simulink model "SPGF_FSK_0000_R2019b"  (R2019b)
settings: Solver=ode3  SolverName=ode4  StartTime=0.0  StopTime=1.4  FixedStep=50e-6/50  RelTol=1e-3  EnableMultiTasking=on
undefined symbols (not defined in the file): D11, Delta
libraries: powerlib x2544, powerlib_meascontrol x204, simulink x24
(part 12 of 33)

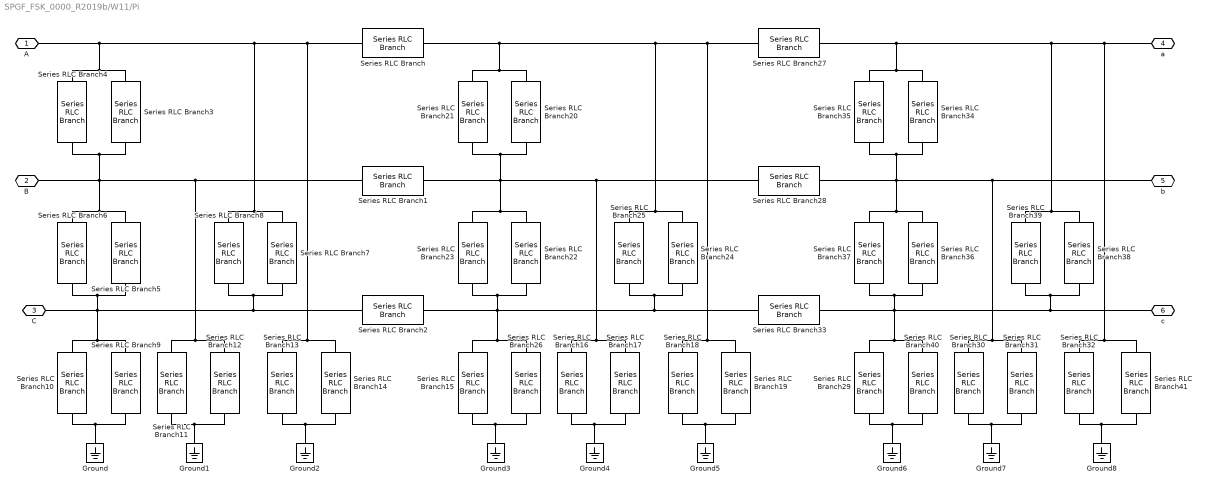
== system SPGF_FSK_0000_R2019b/W11/Pi ==
  Ground{,1..8} (9 alike) : powerlib/Elements/Ground  LConnTagsString=a
  Series RLC Branch{,1..2,27..28,33} (6 alike) : powerlib/Elements/Series RLC Branch  LConnTagsString=__new0  RConnTagsString=__new0  BranchType=RL  Resistance=R/2  Inductance=L/2  SetiL0=off  InitialCurrent=0  Capacitance=1e-6  Setx0=off  InitialVoltage=0  Measurements=None
  Series RLC Branch{10..11,13,29..30,32} (6 alike) : powerlib/Elements/Series RLC Branch  LConnTagsString=__new0  RConnTagsString=__new0  BranchType=R  Resistance=Rfg*4  Inductance=L/2  SetiL0=off  InitialCurrent=0  Capacitance=1e-6  Setx0=off  InitialVoltage=0  Measurements=None
  Series RLC Branch{9,12,14,31,40..41} (6 alike) : powerlib/Elements/Series RLC Branch  LConnTagsString=__new0  RConnTagsString=__new0  BranchType=C  Resistance=R/2  Inductance=L/2  SetiL0=off  InitialCurrent=0  Capacitance=Cfg*0.25  Setx0=off  InitialVoltage=0  Measurements=None
  Series RLC Branch15 : powerlib/Elements/Series RLC Branch  LConnTagsString=__new0  RConnTagsString=__new0  BranchType=R  Resistance=Rfg*2  Inductance=L/2  SetiL0=off  InitialCurrent=0  Capacitance=1e-6  Setx0=off  InitialVoltage=0  Measurements=None
  Series RLC Branch16 : powerlib/Elements/Series RLC Branch  LConnTagsString=__new0  RConnTagsString=__new0  BranchType=R  Resistance=Rfg*2  Inductance=L/2  SetiL0=off  InitialCurrent=0  Capacitance=1e-6  Setx0=off  InitialVoltage=0  Measurements=None
  Series RLC Branch17 : powerlib/Elements/Series RLC Branch  LConnTagsString=__new0  RConnTagsString=__new0  BranchType=C  Resistance=R/2  Inductance=L/2  SetiL0=off  InitialCurrent=0  Capacitance=Cfg*0.5  Setx0=off  InitialVoltage=0  Measurements=None
  Series RLC Branch18 : powerlib/Elements/Series RLC Branch  LConnTagsString=__new0  RConnTagsString=__new0  BranchType=R  Resistance=Rfg*2  Inductance=L/2  SetiL0=off  InitialCurrent=0  Capacitance=1e-6  Setx0=off  InitialVoltage=0  Measurements=None
  Series RLC Branch19 : powerlib/Elements/Series RLC Branch  LConnTagsString=__new0  RConnTagsString=__new0  BranchType=C  Resistance=R/2  Inductance=L/2  SetiL0=off  InitialCurrent=0  Capacitance=Cfg*0.5  Setx0=off  InitialVoltage=0  Measurements=None
  Series RLC Branch20 : powerlib/Elements/Series RLC Branch  LConnTagsString=__new0  RConnTagsString=__new0  BranchType=C  Resistance=R/2  Inductance=L/2  SetiL0=off  InitialCurrent=0  Capacitance=Cmf*0.5  Setx0=off  InitialVoltage=0  Measurements=None
  Series RLC Branch21 : powerlib/Elements/Series RLC Branch  LConnTagsString=__new0  RConnTagsString=__new0  BranchType=R  Resistance=Rmf*2  Inductance=L/2  SetiL0=off  InitialCurrent=0  Capacitance=1e-6  Setx0=off  InitialVoltage=0  Measurements=None
  Series RLC Branch22 : powerlib/Elements/Series RLC Branch  LConnTagsString=__new0  RConnTagsString=__new0  BranchType=C  Resistance=R/2  Inductance=L/2  SetiL0=off  InitialCurrent=0  Capacitance=Cmf*0.5  Setx0=off  InitialVoltage=0  Measurements=None
  Series RLC Branch23 : powerlib/Elements/Series RLC Branch  LConnTagsString=__new0  RConnTagsString=__new0  BranchType=R  Resistance=Rmf*2  Inductance=L/2  SetiL0=off  InitialCurrent=0  Capacitance=1e-6  Setx0=off  InitialVoltage=0  Measurements=None
  Series RLC Branch24 : powerlib/Elements/Series RLC Branch  LConnTagsString=__new0  RConnTagsString=__new0  BranchType=C  Resistance=R/2  Inductance=L/2  SetiL0=off  InitialCurrent=0  Capacitance=Cmf*0.5  Setx0=off  InitialVoltage=0  Measurements=None
  Series RLC Branch25 : powerlib/Elements/Series RLC Branch  LConnTagsString=__new0  RConnTagsString=__new0  BranchType=R  Resistance=Rmf*2  Inductance=L/2  SetiL0=off  InitialCurrent=0  Capacitance=1e-6  Setx0=off  InitialVoltage=0  Measurements=None
  Series RLC Branch26 : powerlib/Elements/Series RLC Branch  LConnTagsString=__new0  RConnTagsString=__new0  BranchType=C  Resistance=R/2  Inductance=L/2  SetiL0=off  InitialCurrent=0  Capacitance=Cfg*0.5  Setx0=off  InitialVoltage=0  Measurements=None
  Series RLC Branch{3,5,7,34,36,38} (6 alike) : powerlib/Elements/Series RLC Branch  LConnTagsString=__new0  RConnTagsString=__new0  BranchType=C  Resistance=R/2  Inductance=L/2  SetiL0=off  InitialCurrent=0  Capacitance=Cmf*0.25  Setx0=off  InitialVoltage=0  Measurements=None
  Series RLC Branch{4,6,8,35,37,39} (6 alike) : powerlib/Elements/Series RLC Branch  LConnTagsString=__new0  RConnTagsString=__new0  BranchType=R  Resistance=Rmf*4  Inductance=L/2  SetiL0=off  InitialCurrent=0  Capacitance=1e-6  Setx0=off  InitialVoltage=0  Measurements=None
  A : PMIOPort  Side=Left
  B : PMIOPort  Port=2  Side=Left
  C : PMIOPort  Port=3  Side=Left
  a : PMIOPort  Port=4  Side=Right
  b : PMIOPort  Port=5  Side=Right
  c : PMIOPort  Port=6  Side=Right
  connections:
  Series RLC Branch12/LConn1 -- Series RLC Branch11/LConn1 -- Series RLC Branch5/LConn1 -- Series RLC Branch6/LConn1 -- B/RConn1 -- Series RLC Branch4/RConn1 -- Series RLC Branch3/RConn1 -- Series RLC Branch1/LConn1
  Series RLC Branch13/LConn1 -- A/RConn1 -- Series RLC Branch4/LConn1 -- Series RLC Branch3/LConn1 -- Series RLC Branch7/LConn1 -- Series RLC Branch8/LConn1 -- Series RLC Branch/LConn1 -- Series RLC Branch14/LConn1
  Series RLC Branch9/LConn1 -- Series RLC Branch2/LConn1 -- Series RLC Branch8/RConn1 -- Series RLC Branch7/RConn1 -- C/RConn1 -- Series RLC Branch5/RConn1 -- Series RLC Branch6/RConn1 -- Series RLC Branch10/LConn1
  Series RLC Branch9/RConn1 -- Ground/LConn1 -- Series RLC Branch10/RConn1
  Series RLC Branch12/RConn1 -- Series RLC Branch11/RConn1 -- Ground1/LConn1
  Series RLC Branch13/RConn1 -- Series RLC Branch14/RConn1 -- Ground2/LConn1
  Series RLC Branch17/LConn1 -- Series RLC Branch16/LConn1 -- Series RLC Branch28/LConn1 -- Series RLC Branch1/RConn1 -- Series RLC Branch23/LConn1 -- Series RLC Branch22/LConn1 -- Series RLC Branch20/RConn1 -- Series RLC Branch21/RConn1
  Series RLC Branch21/LConn1 -- Series RLC Branch20/LConn1 -- Series RLC Branch/RConn1 -- Series RLC Branch27/LConn1 -- Series RLC Branch19/LConn1 -- Series RLC Branch18/LConn1 -- Series RLC Branch24/LConn1 -- Series RLC Branch25/LConn1
  Series RLC Branch26/LConn1 -- Series RLC Branch15/LConn1 -- Series RLC Branch2/RConn1 -- Series RLC Branch33/LConn1 -- Series RLC Branch25/RConn1 -- Series RLC Branch24/RConn1 -- Series RLC Branch22/RConn1 -- Series RLC Branch23/RConn1
  Series RLC Branch26/RConn1 -- Series RLC Branch15/RConn1 -- Ground3/LConn1
  Ground4/LConn1 -- Series RLC Branch17/RConn1 -- Series RLC Branch16/RConn1
  Ground5/LConn1 -- Series RLC Branch18/RConn1 -- Series RLC Branch19/RConn1
  Series RLC Branch31/LConn1 -- b/RConn1 -- Series RLC Branch35/RConn1 -- Series RLC Branch34/RConn1 -- Series RLC Branch36/LConn1 -- Series RLC Branch37/LConn1 -- Series RLC Branch28/RConn1 -- Series RLC Branch30/LConn1
  Series RLC Branch34/LConn1 -- a/RConn1 -- Series RLC Branch41/LConn1 -- Series RLC Branch32/LConn1 -- Series RLC Branch38/LConn1 -- Series RLC Branch39/LConn1 -- Series RLC Branch27/RConn1 -- Series RLC Branch35/LConn1
  Series RLC Branch29/LConn1 -- Series RLC Branch36/RConn1 -- Series RLC Branch37/RConn1 -- c/RConn1 -- Series RLC Branch39/RConn1 -- Series RLC Branch38/RConn1 -- Series RLC Branch33/RConn1 -- Series RLC Branch40/LConn1
  Series RLC Branch29/RConn1 -- Series RLC Branch40/RConn1 -- Ground6/LConn1
  Series RLC Branch31/RConn1 -- Series RLC Branch30/RConn1 -- Ground7/LConn1
  Series RLC Branch32/RConn1 -- Series RLC Branch41/RConn1 -- Ground8/LConn1

== system SPGF_FSK_0000_R2019b/W11/Q ==
  breaker : Subsystem  Commented=on  mask{SwitchA=on, SwitchB=on, SwitchC=on, InitialStatus=[0 0 0], BreakerResistance=0.0001, SnubberResistance=1e6, SnubberCapacitance=inf, TransitionTimes=[0.2], ShiftTimes=[0 0.02 0.04]}
      mask prompts: SwitchA "Switching of phase A"; SwitchB "Switching of phase B"; SwitchC "Switching of phase C"; InitialStatus "Initial status of phase breaker [A, B, C]"; BreakerResistance "Breaker resistance Ron (ohms) :"; SnubberResistance "Snubbers resistance Rp (ohms) :"; SnubberCapacitance "Snubbers capacitance Cp (F) :"; TransitionTimes "Transition times (s) :"; ShiftTimes "Time differences for switch [tA, tB, tC] (s) :"
      mask init: same as SPGF_FSK_0000_R2019b/Feed/Q/breaker
      mask Display:
      | % port_label('input',1,'Iabc');
      | 
      | port_label('lconn',1,'A');
      | port_label('lconn',2,'B');
      | port_label('lconn',3,'C');
      | 
      | port_label('rconn',1,'a');
      | port_label('rconn',2,'b');
      | port_label('rconn',3,'c');
      | 
      | disp('   Q    ');
  meas : Subsystem
  shunt : Subsystem
  A : PMIOPort  Side=Right
  B : PMIOPort  Port=2  Side=Right
  C : PMIOPort  Port=3  Side=Right
  a : PMIOPort  Port=4  Side=Left
  b : PMIOPort  Port=5  Side=Left
  c : PMIOPort  Port=6  Side=Left
  connections:
  shunt/LConn3 -- breaker/LConn3 -- C/RConn1
  shunt/LConn2 -- breaker/LConn2 -- B/RConn1
  A/RConn1 -- breaker/LConn1 -- shunt/LConn1
  meas/RConn1 -- a/RConn1
  meas/RConn2 -- b/RConn1
  meas/RConn3 -- c/RConn1
  breaker/RConn3 -- shunt/RConn3 -- meas/LConn3
  breaker/RConn2 -- shunt/RConn2 -- meas/LConn2
  breaker/RConn1 -- shunt/RConn1 -- meas/LConn1

== system SPGF_FSK_0000_R2019b/W11/concentrated ==
  Ccs/1 : powerlib/Elements/Series RLC Branch  LConnTagsString=__new0  RConnTagsString=__new0  BranchType=C  Resistance=190  Inductance=1e-3  SetiL0=off  InitialCurrent=0  Capacitance=-C_matrix(1,2)/2  Setx0=off  InitialVoltage=0  Measurements=None
  Ccs/2 : powerlib/Elements/Series RLC Branch  LConnTagsString=__new0  RConnTagsString=__new0  BranchType=C  Resistance=190  Inductance=1e-3  SetiL0=off  InitialCurrent=0  Capacitance=-C_matrix(1,2)/2  Setx0=off  InitialVoltage=0  Measurements=None
  Ccs2/1 : powerlib/Elements/Series RLC Branch  LConnTagsString=__new0  RConnTagsString=__new0  BranchType=C  Resistance=190  Inductance=1e-3  SetiL0=off  InitialCurrent=0  Capacitance=-C_matrix(3,4)/2  Setx0=off  InitialVoltage=0  Measurements=None
  Ccs2/2 : powerlib/Elements/Series RLC Branch  LConnTagsString=__new0  RConnTagsString=__new0  BranchType=C  Resistance=190  Inductance=1e-3  SetiL0=off  InitialCurrent=0  Capacitance=-C_matrix(3,4)/2  Setx0=off  InitialVoltage=0  Measurements=None
  Ccs2/3 : powerlib/Elements/Series RLC Branch  LConnTagsString=__new0  RConnTagsString=__new0  BranchType=R  Resistance=-Rg_matrix(3,4)*2  Inductance=1e-3  SetiL0=off  InitialCurrent=0  Capacitance=Rg_matrix(3,4)*2  Setx0=off  InitialVoltage=0  Measurements=None
  Ccs2/4 : powerlib/Elements/Series RLC Branch  LConnTagsString=__new0  RConnTagsString=__new0  BranchType=R  Resistance=-Rg_matrix(3,4)*2  Inductance=1e-3  SetiL0=off  InitialCurrent=0  Capacitance=Rg_matrix(3,4)*2  Setx0=off  InitialVoltage=0  Measurements=None
  Ccs3/1 : powerlib/Elements/Series RLC Branch  LConnTagsString=__new0  RConnTagsString=__new0  BranchType=C  Resistance=190  Inductance=1e-3  SetiL0=off  InitialCurrent=0  Capacitance=-C_matrix(5,6)/2  Setx0=off  InitialVoltage=0  Measurements=None
  Ccs3/2 : powerlib/Elements/Series RLC Branch  LConnTagsString=__new0  RConnTagsString=__new0  BranchType=C  Resistance=190  Inductance=1e-3  SetiL0=off  InitialCurrent=0  Capacitance=-C_matrix(5,6)/2  Setx0=off  InitialVoltage=0  Measurements=None
  Ccs3/3 : powerlib/Elements/Series RLC Branch  LConnTagsString=__new0  RConnTagsString=__new0  BranchType=R  Resistance=-Rg_matrix(5,6)*2  Inductance=1e-3  SetiL0=off  InitialCurrent=0  Capacitance=-C_matrix(5,6)/2  Setx0=off  InitialVoltage=0  Measurements=None
  Ccs3/4 : powerlib/Elements/Series RLC Branch  LConnTagsString=__new0  RConnTagsString=__new0  BranchType=R  Resistance=-Rg_matrix(5,6)*2  Inductance=1e-3  SetiL0=off  InitialCurrent=0  Capacitance=-C_matrix(5,6)/2  Setx0=off  InitialVoltage=0  Measurements=None
  Csg/2 : powerlib/Elements/Series RLC Branch  LConnTagsString=__new0  RConnTagsString=__new0  BranchType=C  Resistance=190  Inductance=1e-3  SetiL0=off  InitialCurrent=0  Capacitance=( C_matrix(1,2) + C_matrix(2,2) )/2  Setx0=off  InitialVoltage=0  Measurements=None
  Csg1/1 : powerlib/Elements/Series RLC Branch  LConnTagsString=__new0  RConnTagsString=__new0  BranchType=C  Resistance=190  Inductance=1e-3  SetiL0=off  InitialCurrent=0  Capacitance=( C_matrix(1,2) + C_matrix(2,2) )/2  Setx0=off  InitialVoltage=0  Measurements=None
  Csg2/1 : powerlib/Elements/Series RLC Branch  LConnTagsString=__new0  RConnTagsString=__new0  BranchType=C  Resistance=190  Inductance=1e-3  SetiL0=off  InitialCurrent=0  Capacitance=( C_matrix(3,4) + C_matrix(4,4) )/2  Setx0=off  InitialVoltage=0  Measurements=None
  Csg2/2 : powerlib/Elements/Series RLC Branch  LConnTagsString=__new0  RConnTagsString=__new0  BranchType=C  Resistance=190  Inductance=1e-3  SetiL0=off  InitialCurrent=0  Capacitance=( C_matrix(3,4) + C_matrix(4,4) )/2  Setx0=off  InitialVoltage=0  Measurements=None
  Csg3/1 : powerlib/Elements/Series RLC Branch  LConnTagsString=__new0  RConnTagsString=__new0  BranchType=C  Resistance=190  Inductance=1e-3  SetiL0=off  InitialCurrent=0  Capacitance=( C_matrix(5,6) + C_matrix(6,6) ) /2  Setx0=off  InitialVoltage=0  Measurements=None
  Csg3/2 : powerlib/Elements/Series RLC Branch  LConnTagsString=__new0  RConnTagsString=__new0  BranchType=C  Resistance=190  Inductance=1e-3  SetiL0=off  InitialCurrent=0  Capacitance=( C_matrix(5,6) + C_matrix(6,6) ) /2  Setx0=off  InitialVoltage=0  Measurements=None
  Ground{1..4} (4 alike) : powerlib/Elements/Ground  LConnTagsString=a
  RL : powerlib/Elements/Mutual Inductance  LConnTagsString=a|b|c|L4|L5|L6  RConnTagsString=A|B|C|R4|R5|R6  TypeOfMutual=Generalized mutual inductance  NumberOfWindings=6  SelfImpedance1=[1.1 1.1e-03]  SelfImpedance2=[ 1.1 1.1e-03]  ThreeWindings=on  SelfImpedance3=[ 1.1 1.1e-03]  MutualImpedance=[1.0 1.0e-03]  InductanceMatrix=L_matrix  ResistanceMatrix=R_matrix  Measurements=None
      settings: AttributesFormatString=\n
  Rcs*2 : powerlib/Elements/Series RLC Branch  LConnTagsString=__new0  RConnTagsString=__new0  BranchType=R  Resistance=-Rg_matrix(1,2)*2  Inductance=1e-3  SetiL0=off  InitialCurrent=0  Capacitance=Rg_matrix(1,2)*2  Setx0=off  InitialVoltage=0  Measurements=None
  Rgcs1/1 : powerlib/Elements/Series RLC Branch  LConnTagsString=__new0  RConnTagsString=__new0  BranchType=R  Resistance=-Rg_matrix(1,2)*2  Inductance=1e-3  SetiL0=off  InitialCurrent=0  Capacitance=Rg_matrix(1,2)*2  Setx0=off  InitialVoltage=0  Measurements=None
  Rgsg1/1 : powerlib/Elements/Series RLC Branch  LConnTagsString=__new0  RConnTagsString=__new0  BranchType=R  Resistance=(Rg_matrix(4,4)+Rg_matrix(3,4))*2  Inductance=1e-3  SetiL0=off  InitialCurrent=0  Capacitance=Rg_matrix(1,2)*2  Setx0=off  InitialVoltage=0  Measurements=None
  Rgsg1/2 : powerlib/Elements/Series RLC Branch  LConnTagsString=__new0  RConnTagsString=__new0  BranchType=R  Resistance=(Rg_matrix(2,2)+Rg_matrix(1,2))*2  Inductance=1e-3  SetiL0=off  InitialCurrent=0  Capacitance=Rg_matrix(1,2)*2  Setx0=off  InitialVoltage=0  Measurements=None
  Rgsg1/3 : powerlib/Elements/Series RLC Branch  LConnTagsString=__new0  RConnTagsString=__new0  BranchType=R  Resistance=(Rg_matrix(4,4)+Rg_matrix(3,4))*2  Inductance=1e-3  SetiL0=off  InitialCurrent=0  Capacitance=Rg_matrix(1,2)*2  Setx0=off  InitialVoltage=0  Measurements=None
  Rgsg1/4 : powerlib/Elements/Series RLC Branch  LConnTagsString=__new0  RConnTagsString=__new0  BranchType=R  Resistance=(Rg_matrix(2,2)+Rg_matrix(1,2))*2  Inductance=1e-3  SetiL0=off  InitialCurrent=0  Capacitance=Rg_matrix(1,2)*2  Setx0=off  InitialVoltage=0  Measurements=None
  Rsg*2 : powerlib/Elements/Series RLC Branch  LConnTagsString=__new0  RConnTagsString=__new0  BranchType=R  Resistance=(Rg_matrix(6,6)+Rg_matrix(5,6))*2  Inductance=1e-3  SetiL0=off  InitialCurrent=0  Capacitance=Rg_matrix(1,2)*2  Setx0=off  InitialVoltage=0  Measurements=None
  Rsg1/1 : powerlib/Elements/Series RLC Branch  LConnTagsString=__new0  RConnTagsString=__new0  BranchType=R  Resistance=(Rg_matrix(6,6)+Rg_matrix(5,6))*2  Inductance=1e-3  SetiL0=off  InitialCurrent=0  Capacitance=Rg_matrix(1,2)*2  Setx0=off  InitialVoltage=0  Measurements=None
  A : PMIOPort  Side=Left
  B : PMIOPort  Port=2  Side=Left
  C : PMIOPort  Port=3  Side=Left
  a : PMIOPort  Port=4  Side=Right
  b : PMIOPort  Port=5  Side=Right
  c : PMIOPort  Port=6  Side=Right
  connections:
  RL/LConn5 -- Ccs3/2/RConn1 -- Ccs3/3/RConn1 -- C/RConn1
  RL/LConn3 -- Ccs2/2/RConn1 -- Ccs2/3/RConn1 -- B/RConn1
  RL/LConn1 -- Ccs/2/RConn1 -- Rcs*2/RConn1 -- A/RConn1
  RL/RConn5 -- Ccs3/1/RConn1 -- Ccs3/4/RConn1 -- c/RConn1
  RL/RConn3 -- Ccs2/1/RConn1 -- Ccs2/4/RConn1 -- b/RConn1
  RL/RConn1 -- Ccs/1/RConn1 -- Rgcs1/1/RConn1 -- a/RConn1
  Csg/2/RConn1 -- Ground1/LConn1 -- Csg3/2/RConn1 -- Rgsg1/2/RConn1 -- Rgsg1/1/RConn1 -- Rsg*2/RConn1 -- Csg2/2/RConn1
  Ccs3/4/LConn1 -- Ccs3/1/LConn1 -- RL/RConn6 -- RL/RConn2 -- Csg1/1/LConn1 -- Rgcs1/1/LConn1 -- Rgsg1/4/LConn1 -- Ccs/1/LConn1 -- RL/RConn4 -- Ccs2/1/LConn1 -- Csg2/1/LConn1 -- Ccs2/4/LConn1 -- Rgsg1/3/LConn1 -- Ground4/LConn1 -- Rsg1/1/LConn1 -- Csg3/1/LConn1
  Csg1/1/RConn1 -- Ground2/LConn1 -- Csg3/1/RConn1 -- Rgsg1/4/RConn1 -- Rgsg1/3/RConn1 -- Rsg1/1/RConn1 -- Csg2/1/RConn1
  RL/LConn2 -- Ccs/2/LConn1 -- Rcs*2/LConn1 -- Csg/2/LConn1 -- Rgsg1/2/LConn1 -- Ccs2/2/LConn1 -- Ccs2/3/LConn1 -- Csg2/2/LConn1 -- Rgsg1/1/LConn1 -- RL/LConn4 -- Ground3/LConn1 -- Ccs3/2/LConn1 -- Ccs3/3/LConn1 -- Csg3/2/LConn1 -- Rsg*2/LConn1 -- RL/LConn6

== system SPGF_FSK_0000_R2019b/W12/DPL ==
  Ccs2/1 : powerlib/Elements/Series RLC Branch  LConnTagsString=__new0  RConnTagsString=__new0  BranchType=R  Resistance=-Rg_matrix(3,4)*2  Inductance=1e-3  SetiL0=off  InitialCurrent=0  Capacitance=Rg_matrix(3,4)*2  Setx0=off  InitialVoltage=0  Measurements=None
  Ccs2/3 : powerlib/Elements/Series RLC Branch  LConnTagsString=__new0  RConnTagsString=__new0  BranchType=R  Resistance=-Rg_matrix(3,4)*2  Inductance=1e-3  SetiL0=off  InitialCurrent=0  Capacitance=Rg_matrix(3,4)*2  Setx0=off  InitialVoltage=0  Measurements=None
  Ccs3/1 : powerlib/Elements/Series RLC Branch  LConnTagsString=__new0  RConnTagsString=__new0  BranchType=R  Resistance=-Rg_matrix(5,6)*2  Inductance=1e-3  SetiL0=off  InitialCurrent=0  Capacitance=-C_matrix(5,6)/2  Setx0=off  InitialVoltage=0  Measurements=None
  Ccs3/3 : powerlib/Elements/Series RLC Branch  LConnTagsString=__new0  RConnTagsString=__new0  BranchType=R  Resistance=-Rg_matrix(5,6)*2  Inductance=1e-3  SetiL0=off  InitialCurrent=0  Capacitance=-C_matrix(5,6)/2  Setx0=off  InitialVoltage=0  Measurements=None
  DPL : powerlib/Elements/Distributed Parameters Line  Phases=6  Length=LineLength  Frequency=Frequency  Resistance=R_matrix  Inductance=L_matrix  Capacitance=C_matrix  x1=[-5.3e-05 -1.50939355674186 0 0 0 0 -8872.61351094603;-5.25e-05 -1.50980377797187 0 0 0 0 -8871.84731916744;-5.2e-05 -1.51021396194896 0 0 0 0 -8871.0809084848;-5.15e-05 -1.51062410866302 0 0 0 0 -8870.314278917;-5.1e-05 -1.51103421810392 0 0 0 0 -8869.54743048298;-5.05e-05 -1.51144429026155 0 0 0 0 -8868.78036320164;-5e-05 -1.51185432512578 0 0 0 0 -8868.01307709192;-4.95e-05 -1.51226432268651 0 0 0 0 -8867.24557217275;-4.9e-05 -1.5126742829336 0 0 0 0 -8866.47784846306;-4.85e-05 -1.51308420585696 0 0 0 0 -8865.70990598181;-4.8e-05 -1.51349409144646 0 0 0 0 -8864.94174474793;-4.75e-05 -1.51390393969199 0 0 0 0 -8864.17336478037;-4.7e-05 -1.51431375058343 0 0 0 0 -8863.40476609811;-4.65e-05 -1.51472352411069 0 0 0 0 -8862.63594872011;-4.6e-05 -1.51513326026364 0 0 0 0 -8861.86691266532;-4.55e-05 -1.51554295903217 0 0 0 0 -8861.09765795274;-4.5e-05 -1.51595262040618 0 0 0 0 -8860.32818460133;-4.45e-05 -1.51636224437556 0 0 0 0 -8859.55849263009;-4.4e-05 -1.5167718309302 0 0 0 0 -8858.78858205801;-4.35e-05 -1.51718138005999 0 0 0 0 -8858.01845290408;-4.3e-05 -1.51759089175484 0 0 0 0 -8857.2481051873;-4.25e-05 -1.51800036600463 0 0 0 0 -8856.47753892669;-4.2e-05 -1.51840980279926 0 0 0 0 -8855.70675414126;-4.15e-05 -1.51881920212864 0 0 0 0 -8854.93575085002;-4.1e-05 -1.51922856398265 0 0 0 0 -8854.164529072;-4.05e-05 -1.5196378883512 0 0 0 0 -8853.39308882622;-4e-05 -1.52004717522418 0 0 0 0 -8852.62143013173;-3.95e-05 -1.52045642459151 0 0 0 0 -8851.84955300756;-3.9e-05 -1.52086563644308 0 0 0 0 -8851.07745747275;-3.85e-05 -1.52127481076879 0 0 0 0 -8850.30514354637;-3.8e-05 -1.52168394755855 0 0 0 0 -8849.53261124746;-3.75e-05 -1.52209304680227 0 0 0 0 -8848.75986059508;-3.7e-05 -1.52250210848984 0 0 0 0 -8847.9868916083;-3.65e-05 -1.52291113261118 0 0 0 0 -8847.2137043062;-3.6e-05 -1.5233201191562 0 0 0 0 -8846.44029870786;-3.55e-05 -1.5237290681148 0 0 0 0 -8845.66667483234;-3.5e-05 -1.52413797947689 0 0 0 0 -8844.89283269876;-3.45e-05 -1.52454685323238 0 0 0 0 -8844.11877232619;-3.4e-05 -1.52495568937119 0 0 0 0 -8843.34449373373;-3.35e-05 -1.52536448788322 0 0 0 0 -8842.5699969405;-3.3e-05 -1.52577324875839 0 0 0 0 -8841.79528196559;-3.25e-05 -1.52618197198662 0 0 0 0 -8841.02034882814;-3.2e-05 -1.52659065755782 0 0 0 0 -8840.24519754725;-3.15e-05 -1.5269993054619 0 0 0 0 -8839.46982814205;-3.1e-05 -1.52740791568878 0 0 0 0 -8838.69424063168;-3.05e-05 -1.52781648822839 0 0 0 0 -8837.91843503527;-3e-05 -1.52822502307063 0 0 0 0 -8837.14241137197;-2.95e-05 -1.52863352020544 0 0 0 0 -8836.36616966091;-2.9e-05 -1.52904197962272 0 0 0 0 -8835.58970992126;-2.85e-05 -1.52945040131241 0 0 0 0 -8834.81303217217;-2.8e-05 -1.52985878526441 0 0 0 0 -8834.03613643281;-2.75e-05 -1.53026713146867 0 0 0 0 -8833.25902272235;-2.7e-05 -1.5306754399151 0 0 0 0 -8832.48169105995;-2.65e-05 -1.53108371059362 0 0 0 0 -8831.70414146481;-2.6e-05 -1.53149194349417 0 0 0 0 -8830.9263739561;-2.55e-05 -1.53190013860667 0 0 0 0 -8830.14838855301;-2.5e-05 -1.53230829592105 0 0 0 0 -8829.37018527475;-2.45e-05 -1.53271641542724 0 0 0 0 -8828.59176414051;-2.4e-05 -1.53312449711517 0 0 0 0 -8827.8131251695;-2.35e-05 -1.53353254097476 0 0 0 0 -8827.03426838094;-2.3e-05 -1.53394054699596 0 0 0 0 -8826.25519379403;-2.25e-05 -1.53434851516869 0 0 0 0 -8825.475901428;-2.2e-05 -1.53475644548289 0 0 0 0 -8824.69639130209;-2.15e-05 -1.53516433792849 0 0 0 0 -8823.91666343552;-2.1e-05 -1.53557219249543 0 0 0 0 -8823.13671784754;-2.05e-05 -1.53598000917365 0 0 0 0 -8822.35655455738;-2e-05 -1.53638778795308 0 0 0 0 -8821.5761735843;-1.95e-05 -1.53679552882365 0 0 0 0 -8820.79557494756;-1.9e-05 -1.53720323177532 0 0 0 0 -8820.0147586664;-1.85e-05 -1.53761089679802 0 0 0 0 -8819.23372476011;-1.8e-05 -1.53801852388169 0 0 0 0 -8818.45247324795;-1.75e-05 -1.53842611301628 0 0 0 0 -8817.67100414919;-1.7e-05 -1.53883366419172 0 0 0 0 -8816.88931748313;-1.65e-05 -1.53924117739797 0 0 0 0 -8816.10741326904;-1.6e-05 -1.53964865262496 0 0 0 0 -8815.32529152621;-1.55e-05 ...(+2780 chars)]  x2=[-5.3e-05 -1.50564703819446 0 0 0 0 -8948.23948235752;-5.25e-05 -1.50606747011388 0 0 0 0 -8947.47202642379;-5.2e-05 -1.50648786487257 0 0 0 0 -8946.70434972004;-5.15e-05 -1.50690822246016 0 0 0 0 -8945.93645226522;-5.1e-05 -1.50732854286628 0 0 0 0 -8945.16833407825;-5.05e-05 -1.50774882608056 0 0 0 0 -8944.39999517811;-5e-05 -1.50816907209263 0 0 0 0 -8943.63143558374;-4.95e-05 -1.50858928089212 0 0 0 0 -8942.86265531411;-4.9e-05 -1.50900945246867 0 0 0 0 -8942.09365438819;-4.85e-05 -1.50942958681189 0 0 0 0 -8941.32443282496;-4.8e-05 -1.50984968391144 0 0 0 0 -8940.55499064338;-4.75e-05 -1.51026974375693 0 0 0 0 -8939.78532786246;-4.7e-05 -1.51068976633802 0 0 0 0 -8939.01544450117;-4.65e-05 -1.51110975164433 0 0 0 0 -8938.24534057852;-4.6e-05 -1.5115296996655 0 0 0 0 -8937.47501611351;-4.55e-05 -1.51194961039117 0 0 0 0 -8936.70447112514;-4.5e-05 -1.51236948381097 0 0 0 0 -8935.93370563242;-4.45e-05 -1.51278931991456 0 0 0 0 -8935.16271965438;-4.4e-05 -1.51320911869157 0 0 0 0 -8934.39151321004;-4.35e-05 -1.51362888013164 0 0 0 0 -8933.62008631842;-4.3e-05 -1.51404860422441 0 0 0 0 -8932.84843899856;-4.25e-05 -1.51446829095953 0 0 0 0 -8932.0765712695;-4.2e-05 -1.51488794032664 0 0 0 0 -8931.30448315029;-4.15e-05 -1.5153075523154 0 0 0 0 -8930.53217465997;-4.1e-05 -1.51572712691543 0 0 0 0 -8929.75964581761;-4.05e-05 -1.5161466641164 0 0 0 0 -8928.98689664226;-4e-05 -1.51656616390795 0 0 0 0 -8928.21392715298;-3.95e-05 -1.51698562627973 0 0 0 0 -8927.44073736886;-3.9e-05 -1.51740505122139 0 0 0 0 -8926.66732730897;-3.85e-05 -1.51782443872258 0 0 0 0 -8925.89369699239;-3.8e-05 -1.51824378877296 0 0 0 0 -8925.11984643821;-3.75e-05 -1.51866310136217 0 0 0 0 -8924.34577566553;-3.7e-05 -1.51908237647987 0 0 0 0 -8923.57148469344;-3.65e-05 -1.51950161411571 0 0 0 0 -8922.79697354105;-3.6e-05 -1.51992081425936 0 0 0 0 -8922.02224222747;-3.55e-05 -1.52033997690046 0 0 0 0 -8921.24729077181;-3.5e-05 -1.52075910202868 0 0 0 0 -8920.4721191932;-3.45e-05 -1.52117818963367 0 0 0 0 -8919.69672751077;-3.4e-05 -1.52159723970509 0 0 0 0 -8918.92111574364;-3.35e-05 -1.52201625223261 0 0 0 0 -8918.14528391096;-3.3e-05 -1.52243522720588 0 0 0 0 -8917.36923203185;-3.25e-05 -1.52285416461457 0 0 0 0 -8916.59296012548;-3.2e-05 -1.52327306444834 0 0 0 0 -8915.81646821101;-3.15e-05 -1.52369192669685 0 0 0 0 -8915.03975630757;-3.1e-05 -1.52411075134977 0 0 0 0 -8914.26282443435;-3.05e-05 -1.52452953839676 0 0 0 0 -8913.48567261051;-3e-05 -1.5249482878275 0 0 0 0 -8912.70830085523;-2.95e-05 -1.52536699963164 0 0 0 0 -8911.93070918768;-2.9e-05 -1.52578567379886 0 0 0 0 -8911.15289762706;-2.85e-05 -1.52620431031883 0 0 0 0 -8910.37486619256;-2.8e-05 -1.52662290918122 0 0 0 0 -8909.59661490336;-2.75e-05 -1.5270414703757 0 0 0 0 -8908.81814377869;-2.7e-05 -1.52745999389194 0 0 0 0 -8908.03945283773;-2.65e-05 -1.52787847971962 0 0 0 0 -8907.26054209972;-2.6e-05 -1.5282969278484 0 0 0 0 -8906.48141158386;-2.55e-05 -1.52871533826797 0 0 0 0 -8905.70206130938;-2.5e-05 -1.529133710968 0 0 0 0 -8904.92249129551;-2.45e-05 -1.52955204593817 0 0 0 0 -8904.14270156148;-2.4e-05 -1.52997034316816 0 0 0 0 -8903.36269212654;-2.35e-05 -1.53038860264764 0 0 0 0 -8902.58246300993;-2.3e-05 -1.53080682436629 0 0 0 0 -8901.80201423091;-2.25e-05 -1.5312250083138 0 0 0 0 -8901.02134580872;-2.2e-05 -1.53164315447985 0 0 0 0 -8900.24045776264;-2.15e-05 -1.53206126285412 0 0 0 0 -8899.45935011192;-2.1e-05 -1.53247933342629 0 0 0 0 -8898.67802287585;-2.05e-05 -1.53289736618605 0 0 0 0 -8897.8964760737;-2e-05 -1.53331536112309 0 0 0 0 -8897.11470972475;-1.95e-05 -1.53373331822708 0 0 0 0 -8896.3327238483;-1.9e-05 -1.53415123748772 0 0 0 0 -8895.55051846364;-1.85e-05 -1.5345691188947 0 0 0 0 -8894.76809359006;-1.8e-05 -1.5349869624377 0 0 0 0 -8893.98544924688;-1.75e-05 -1.53540476810641 0 0 0 0 -8893.20258545341;-1.7e-05 -1.53582253589054 0 0 0 0 -8892.41950222896;-1.65e-05 -1.53624026577976 0 0 0 0 -8891.63619959285;-1.6e-05 -1.53665795776377 0 0 0 0 -8890.85267756441;-1.55e-05 ...(+2786 chars)]  x3=[-5.3e-05 0.0131139201948921 0 0 0 0 -275.39648268413;-5.25e-05 0.0131100972254946 0 0 0 0 -275.39032083345;-5.2e-05 0.0131062739326184 0 0 0 0 -275.384152187786;-5.15e-05 0.0131024503163578 0 0 0 0 -275.37797674729;-5.1e-05 0.0130986263768073 0 0 0 0 -275.371794512115;-5.05e-05 0.013094802114061 0 0 0 0 -275.365605482414;-5e-05 0.0130909775282135 0 0 0 0 -275.359409658338;-4.95e-05 0.0130871526193591 0 0 0 0 -275.353207040042;-4.9e-05 0.0130833273875921 0 0 0 0 -275.346997627677;-4.85e-05 0.013079501833007 0 0 0 0 -275.340781421397;-4.8e-05 0.0130756759556981 0 0 0 0 -275.334558421356;-4.75e-05 0.0130718497557598 0 0 0 0 -275.328328627708;-4.7e-05 0.0130680232332866 0 0 0 0 -275.322092040605;-4.65e-05 0.0130641963883728 0 0 0 0 -275.315848660201;-4.6e-05 0.0130603692211129 0 0 0 0 -275.309598486652;-4.55e-05 0.0130565417316013 0 0 0 0 -275.30334152011;-4.5e-05 0.0130527139199324 0 0 0 0 -275.297077760731;-4.45e-05 0.0130488857862007 0 0 0 0 -275.290807208668;-4.4e-05 0.0130450573305007 0 0 0 0 -275.284529864077;-4.35e-05 0.0130412285529268 0 0 0 0 -275.278245727113;-4.3e-05 0.0130373994535735 0 0 0 0 -275.27195479793;-4.25e-05 0.0130335700325352 0 0 0 0 -275.265657076684;-4.2e-05 0.0130297402899065 0 0 0 0 -275.25935256353;-4.15e-05 0.0130259102257818 0 0 0 0 -275.253041258624;-4.1e-05 0.0130220798402557 0 0 0 0 -275.246723162122;-4.05e-05 0.0130182491334227 0 0 0 0 -275.240398274178;-4e-05 0.0130144181053772 0 0 0 0 -275.23406659495;-3.95e-05 0.0130105867562138 0 0 0 0 -275.227728124594;-3.9e-05 0.0130067550860271 0 0 0 0 -275.221382863266;-3.85e-05 0.0130029230949115 0 0 0 0 -275.215030811122;-3.8e-05 0.0129990907829617 0 0 0 0 -275.20867196832;-3.75e-05 0.0129952581502722 0 0 0 0 -275.202306335015;-3.7e-05 0.0129914251969375 0 0 0 0 -275.195933911367;-3.65e-05 0.0129875919230523 0 0 0 0 -275.18955469753;-3.6e-05 0.0129837583287111 0 0 0 0 -275.183168693664;-3.55e-05 0.0129799244140084 0 0 0 0 -275.176775899925;-3.5e-05 0.012976090179039 0 0 0 0 -275.170376316471;-3.45e-05 0.0129722556238974 0 0 0 0 -275.16396994346;-3.4e-05 0.0129684207486782 0 0 0 0 -275.157556781051;-3.35e-05 0.0129645855534761 0 0 0 0 -275.151136829401;-3.3e-05 0.0129607500383856 0 0 0 0 -275.144710088668;-3.25e-05 0.0129569142035015 0 0 0 0 -275.138276559013;-3.2e-05 0.0129530780489183 0 0 0 0 -275.131836240592;-3.15e-05 0.0129492415747307 0 0 0 0 -275.125389133566;-3.1e-05 0.0129454047810334 0 0 0 0 -275.118935238092;-3.05e-05 0.012941567667921 0 0 0 0 -275.112474554331;-3e-05 0.0129377302354883 0 0 0 0 -275.106007082442;-2.95e-05 0.0129338924838298 0 0 0 0 -275.099532822584;-2.9e-05 0.0129300544130404 0 0 0 0 -275.093051774917;-2.85e-05 0.0129262160232146 0 0 0 0 -275.086563939601;-2.8e-05 0.0129223773144473 0 0 0 0 -275.080069316797;-2.75e-05 0.012918538286833 0 0 0 0 -275.073567906663;-2.7e-05 0.0129146989404666 0 0 0 0 -275.067059709362;-2.65e-05 0.0129108592754428 0 0 0 0 -275.060544725053;-2.6e-05 0.0129070192918563 0 0 0 0 -275.054022953897;-2.55e-05 0.0129031789898019 0 0 0 0 -275.047494396055;-2.5e-05 0.0128993383693743 0 0 0 0 -275.040959051688;-2.45e-05 0.0128954974306682 0 0 0 0 -275.034416920957;-2.4e-05 0.0128916561737786 0 0 0 0 -275.027868004024;-2.35e-05 0.0128878145988 0 0 0 0 -275.021312301051;-2.3e-05 0.0128839727058274 0 0 0 0 -275.014749812199;-2.25e-05 0.0128801304949555 0 0 0 0 -275.008180537629;-2.2e-05 0.0128762879662791 0 0 0 0 -275.001604477505;-2.15e-05 0.0128724451198931 0 0 0 0 -274.995021631989;-2.1e-05 0.0128686019558922 0 0 0 0 -274.988432001242;-2.05e-05 0.0128647584743712 0 0 0 0 -274.981835585427;-2e-05 0.0128609146754251 0 0 0 0 -274.975232384708;-1.95e-05 0.0128570705591486 0 0 0 0 -274.968622399247;-1.9e-05 0.0128532261256367 0 0 0 0 -274.962005629207;-1.85e-05 0.0128493813749841 0 0 0 0 -274.955382074751;-1.8e-05 0.0128455363072857 0 0 0 0 -274.948751736044;-1.75e-05 0.0128416909226364 0 0 0 0 -274.942114613248;-1.7e-05 0.0128378452211311 0 0 0 0 -274.935470706527;-1.65e-05 0.0128339992028646 0 0 0 0 ...(+2915 chars)]  x4=[-5.3e-05 -0.0324808035916861 0 0 0 0 14.9886458211936;-5.25e-05 -0.0324824208637865 0 0 0 0 15.004831786322;-5.2e-05 -0.0324840373344152 0 0 0 0 15.021017381221;-5.15e-05 -0.0324856530035325 0 0 0 0 15.0372026054913;-5.1e-05 -0.0324872678710983 0 0 0 0 15.0533874587335;-5.05e-05 -0.032488881937073 0 0 0 0 15.0695719405482;-5e-05 -0.0324904952014167 0 0 0 0 15.0857560505362;-4.95e-05 -0.0324921076640895 0 0 0 0 15.101939788298;-4.9e-05 -0.0324937193250517 0 0 0 0 15.1181231534344;-4.85e-05 -0.0324953301842635 0 0 0 0 15.1343061455461;-4.8e-05 -0.0324969402416852 0 0 0 0 15.1504887642338;-4.75e-05 -0.032498549497277 0 0 0 0 15.1666710090981;-4.7e-05 -0.0325001579509993 0 0 0 0 15.1828528797398;-4.65e-05 -0.0325017656028123 0 0 0 0 15.1990343757596;-4.6e-05 -0.0325033724526763 0 0 0 0 15.2152154967583;-4.55e-05 -0.0325049785005519 0 0 0 0 15.2313962423366;-4.5e-05 -0.0325065837463992 0 0 0 0 15.2475766120953;-4.45e-05 -0.0325081881901787 0 0 0 0 15.2637566056351;-4.4e-05 -0.0325097918318508 0 0 0 0 15.2799362225568;-4.35e-05 -0.032511394671376 0 0 0 0 15.2961154624612;-4.3e-05 -0.0325129967087146 0 0 0 0 15.312294324949;-4.25e-05 -0.0325145979438273 0 0 0 0 15.3284728096212;-4.2e-05 -0.0325161983766743 0 0 0 0 15.3446509160784;-4.15e-05 -0.0325177980072164 0 0 0 0 15.3608286439216;-4.1e-05 -0.0325193968354139 0 0 0 0 15.3770059927515;-4.05e-05 -0.0325209948612275 0 0 0 0 15.3931829621689;-4e-05 -0.0325225920846177 0 0 0 0 15.4093595517749;-3.95e-05 -0.0325241885055451 0 0 0 0 15.4255357611701;-3.9e-05 -0.0325257841239703 0 0 0 0 15.4417115899554;-3.85e-05 -0.0325273789398539 0 0 0 0 15.4578870377318;-3.8e-05 -0.0325289729531567 0 0 0 0 15.4740621041002;-3.75e-05 -0.0325305661638392 0 0 0 0 15.4902367886613;-3.7e-05 -0.0325321585718622 0 0 0 0 15.5064110910162;-3.65e-05 -0.0325337501771864 0 0 0 0 15.5225850107658;-3.6e-05 -0.0325353409797724 0 0 0 0 15.5387585475109;-3.55e-05 -0.0325369309795811 0 0 0 0 15.5549317008525;-3.5e-05 -0.0325385201765732 0 0 0 0 15.5711044703915;-3.45e-05 -0.0325401085707094 0 0 0 0 15.5872768557289;-3.4e-05 -0.0325416961619507 0 0 0 0 15.6034488564657;-3.35e-05 -0.0325432829502578 0 0 0 0 15.6196204722029;-3.3e-05 -0.0325448689355916 0 0 0 0 15.6357917025413;-3.25e-05 -0.032546454117913 0 0 0 0 15.6519625470821;-3.2e-05 -0.0325480384971828 0 0 0 0 15.6681330054261;-3.15e-05 -0.0325496220733619 0 0 0 0 15.6843030771745;-3.1e-05 -0.0325512048464113 0 0 0 0 15.7004727619282;-3.05e-05 -0.0325527868162919 0 0 0 0 15.7166420592883;-3e-05 -0.0325543679829647 0 0 0 0 15.7328109688558;-2.95e-05 -0.0325559483463906 0 0 0 0 15.7489794902317;-2.9e-05 -0.0325575279065307 0 0 0 0 15.7651476230171;-2.85e-05 -0.0325591066633461 0 0 0 0 15.7813153668131;-2.8e-05 -0.0325606846167976 0 0 0 0 15.7974827212208;-2.75e-05 -0.0325622617668465 0 0 0 0 15.8136496858412;-2.7e-05 -0.0325638381134538 0 0 0 0 15.8298162602754;-2.65e-05 -0.0325654136565806 0 0 0 0 15.8459824441246;-2.6e-05 -0.032566988396188 0 0 0 0 15.8621482369898;-2.55e-05 -0.0325685623322372 0 0 0 0 15.8783136384722;-2.5e-05 -0.0325701354646893 0 0 0 0 15.8944786481729;-2.45e-05 -0.0325717077935056 0 0 0 0 15.9106432656931;-2.4e-05 -0.0325732793186471 0 0 0 0 15.9268074906339;-2.35e-05 -0.0325748500400752 0 0 0 0 15.9429713225964;-2.3e-05 -0.0325764199577511 0 0 0 0 15.959134761182;-2.25e-05 -0.0325779890716361 0 0 0 0 15.9752978059916;-2.2e-05 -0.0325795573816914 0 0 0 0 15.9914604566266;-2.15e-05 -0.0325811248878784 0 0 0 0 16.0076227126881;-2.1e-05 -0.0325826915901583 0 0 0 0 16.0237845737774;-2.05e-05 -0.0325842574884925 0 0 0 0 16.0399460394956;-2e-05 -0.0325858225828424 0 0 0 0 16.056107109444;-1.95e-05 -0.0325873868731694 0 0 0 0 16.0722677832238;-1.9e-05 -0.0325889503594348 0 0 0 0 16.0884280604364;-1.85e-05 -0.0325905130416001 0 0 0 0 16.1045879406829;-1.8e-05 -0.0325920749196267 0 0 0 0 16.1207474235646;-1.75e-05 -0.0325936359934761 0 0 0 0 16.1369065086828;-1.7e-05 -0.0325951962631098 0 0 0 0 16.1530651956388;-1.65e-05 -0.0325967557284892 0 0 0 0 ...(+2920 chars)]  x5=5.28312353527576e-05  V1=ones(3,3)  V2=ones(3,3)  I1=ones(3,3)  I2=ones(3,3)  nHarmo=1  Measurements=None  Decoupling=off  VsMag0=0  VrMag0=0  VsAngle0=0  VrAngle0=0  IsMag0=0  IrMag0=0  IsAngle0=0  IrAngle0=0
  Ground{1..4} (4 alike) : powerlib/Elements/Ground  LConnTagsString=a
  Rcs*1 : powerlib/Elements/Series RLC Branch  LConnTagsString=__new0  RConnTagsString=__new0  BranchType=R  Resistance=-Rg_matrix(1,2)*2  Inductance=1e-3  SetiL0=off  InitialCurrent=0  Capacitance=Rg_matrix(1,2)*2  Setx0=off  InitialVoltage=0  Measurements=None
  Rcs*2 : powerlib/Elements/Series RLC Branch  LConnTagsString=__new0  RConnTagsString=__new0  BranchType=R  Resistance=-Rg_matrix(1,2)*2  Inductance=1e-3  SetiL0=off  InitialCurrent=0  Capacitance=Rg_matrix(1,2)*2  Setx0=off  InitialVoltage=0  Measurements=None
  Rgsg1/1 : powerlib/Elements/Series RLC Branch  LConnTagsString=__new0  RConnTagsString=__new0  BranchType=R  Resistance=(Rg_matrix(4,4)+Rg_matrix(3,4))*2  Inductance=1e-3  SetiL0=off  InitialCurrent=0  Capacitance=Rg_matrix(1,2)*2  Setx0=off  InitialVoltage=0  Measurements=None
  Rgsg1/2 : powerlib/Elements/Series RLC Branch  LConnTagsString=__new0  RConnTagsString=__new0  BranchType=R  Resistance=(Rg_matrix(2,2)+Rg_matrix(1,2))*2  Inductance=1e-3  SetiL0=off  InitialCurrent=0  Capacitance=Rg_matrix(1,2)*2  Setx0=off  InitialVoltage=0  Measurements=None
  Rgsg1/3 : powerlib/Elements/Series RLC Branch  LConnTagsString=__new0  RConnTagsString=__new0  BranchType=R  Resistance=(Rg_matrix(4,4)+Rg_matrix(3,4))*2  Inductance=1e-3  SetiL0=off  InitialCurrent=0  Capacitance=Rg_matrix(1,2)*2  Setx0=off  InitialVoltage=0  Measurements=None
  Rgsg1/4 : powerlib/Elements/Series RLC Branch  LConnTagsString=__new0  RConnTagsString=__new0  BranchType=R  Resistance=(Rg_matrix(2,2)+Rg_matrix(1,2))*2  Inductance=1e-3  SetiL0=off  InitialCurrent=0  Capacitance=Rg_matrix(1,2)*2  Setx0=off  InitialVoltage=0  Measurements=None
  Rsg*1 : powerlib/Elements/Series RLC Branch  LConnTagsString=__new0  RConnTagsString=__new0  BranchType=R  Resistance=(Rg_matrix(6,6)+Rg_matrix(5,6))*2  Inductance=1e-3  SetiL0=off  InitialCurrent=0  Capacitance=Rg_matrix(1,2)*2  Setx0=off  InitialVoltage=0  Measurements=None
  Rsg*2 : powerlib/Elements/Series RLC Branch  LConnTagsString=__new0  RConnTagsString=__new0  BranchType=R  Resistance=(Rg_matrix(6,6)+Rg_matrix(5,6))*2  Inductance=1e-3  SetiL0=off  InitialCurrent=0  Capacitance=Rg_matrix(1,2)*2  Setx0=off  InitialVoltage=0  Measurements=None
  A : PMIOPort  Side=Left
  B : PMIOPort  Port=2  Side=Left
  C : PMIOPort  Port=3  Side=Left
  a : PMIOPort  Port=4  Side=Right
  b : PMIOPort  Port=5  Side=Right
  c : PMIOPort  Port=6  Side=Right
  connections:
  A/RConn1 -- DPL/LConn1 -- Rcs*2/RConn1
  B/RConn1 -- DPL/LConn3 -- Ccs2/3/RConn1
  C/RConn1 -- DPL/LConn5 -- Ccs3/3/RConn1
  Rgsg1/2/RConn1 -- Rsg*2/RConn1 -- Rgsg1/1/RConn1 -- Ground2/LConn1
  DPL/LConn2 -- Rcs*2/LConn1 -- Rgsg1/2/LConn1 -- DPL/LConn4 -- Ccs2/3/LConn1 -- Rgsg1/1/LConn1 -- DPL/LConn6 -- Rsg*2/LConn1 -- Ccs3/3/LConn1 -- Ground3/LConn1
  Rgsg1/3/RConn1 -- Rsg*1/RConn1 -- Rgsg1/4/RConn1 -- Ground1/LConn1
  Rgsg1/3/LConn1 -- Ccs2/1/LConn1 -- DPL/RConn4 -- DPL/RConn2 -- Rgsg1/4/LConn1 -- Rcs*1/LConn1 -- Rsg*1/LConn1 -- Ccs3/1/LConn1 -- DPL/RConn6 -- Ground4/LConn1
  Rcs*1/RConn1 -- DPL/RConn1 -- a/RConn1
  DPL/RConn3 -- Ccs2/1/RConn1 -- b/RConn1
  DPL/RConn5 -- Ccs3/1/RConn1 -- c/RConn1
